simulink model "project"  (R2023b)
settings: Solver=VariableStepAuto  StartTime=0.0  StopTime=10.0  RelTol=1e-3
libraries: spsDCVoltageSourceLib x2, spsDCMachineLib x1, sps_lib x1
settings Model: Creator=yasha  LastModifiedBy=yasha

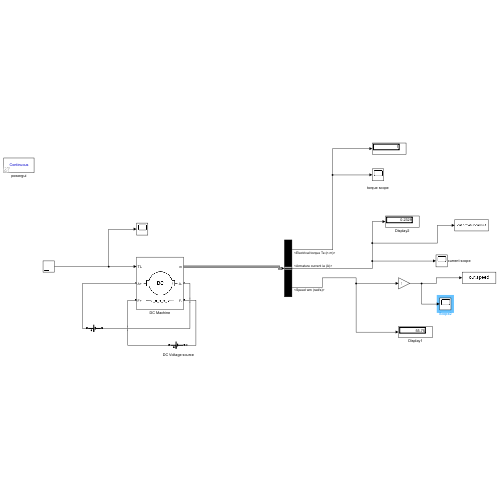
[thumbnail: Simulink's stored preview of the top-level diagram]
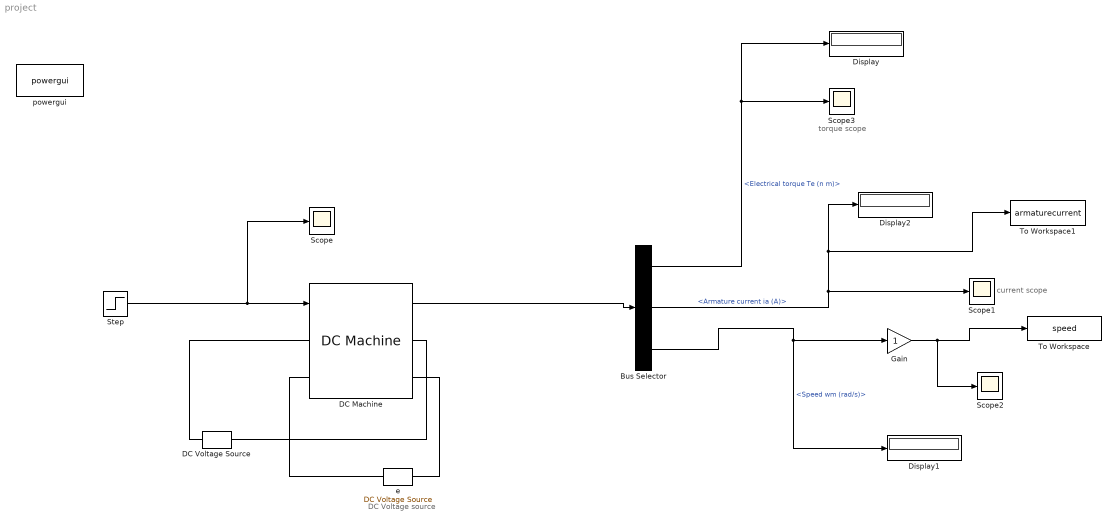
== system project ==
  note: DC Voltage source
  note: current scope
  note: torque scope
  Bus Selector : BusSelector  OutputSignals=Electrical torque Te (n m),Armature current ia (A),Speed wm (rad/s)
  DC Machine : spsDCMachineLib/DC Machine  PresetModel=No  MechanicalLoad=Torque TL  FieldType=Wound  ShowDetailedParameters=on  MeasurementBus=off  RLa=[2.581 0.028]  RLf="[ 53  156]"  Laf=0.9483  MachineConstant=Torque constant (N.m/A)  Ke=1.8  Kt=1.8  J=1  Bm=0  Tf=0  w0=1  Ifinit=4.52830188679245  TsPowergui=0  TsBlock=-1
  DC Voltage Source : spsDCVoltageSourceLib/DC Voltage Source  Amplitude=240  Measurements=None
  Display : Display
  Display1 : Display
  Display2 : Display
  Gain : Gain
  Scope{,1..3} (4 alike) : Scope
  Step : Step  SampleTime=0
  To Workspace : ToWorkspace  VariableName=speed  SaveFormat=Timeseries  SampleTime=-1
  To Workspace1 : ToWorkspace  VariableName=armaturecurrent  SaveFormat=Timeseries  SampleTime=-1
  e : spsDCVoltageSourceLib/DC Voltage Source  Amplitude=240  Measurements=Voltage
  powergui : sps_lib/powergui  Priority=1  SimulationMode=Continuous  SampleTime=50e-6  frequency=60  Iterations=50  frequencyindice=0  Pbase=100e6  ErrMax=1e-4  UnitsV=kV  UnitsW=MW  buscounter=0  FunctionMessages=off  echomessages=off  EnableUseOfTLC=off  CurrentSourceSwitches=off  DisableSnubberDevices=off  DisableRonSwitches=off  DisableVfSwitches=off  DisplayEquations=off  AutomaticDiscreteSolvers=off  SolverType=Tustin/Backward Euler (TBE)  Interpol=off  ExternalGateDelay=off  methode=off  Ts=100  x0status=blocks  SPID=on  SwTol=0  HookPort=off  NonlinearTolerance=1e-4  nMaxIteration=100  ContinueOnMaxIteration=off  RestoreLinks=warning  ResistiveCurrentMeasurement=off  Frange=[0:2:500]  Ylog=off  Xlog=on  ShowGrid=off  save=off  variable=ZData  structure=0  ZoomFFT=off  StartTime=0.0  cycles=1  DisplayStyle=1  fundamental=60  FreqAxis=off  MaxFrequency=1000  frequencyindicesteady=1  RmsSteady=1  display=off
  wires:
  Step/1 -> Scope/1, DC Machine/1
  DC Machine/1 -> Bus Selector/1
  Bus Selector/3 -> Gain/1, Display1/1  "<Speed wm (rad/s)>"
  Bus Selector/1 -> Display/1, Scope3/1  "<Electrical torque Te (n m)>"
  Bus Selector/2 -> To Workspace1/1, Display2/1, Scope1/1  "<Armature current ia (A)>"
  Gain/1 -> Scope2/1, To Workspace/1
  connections:
  DC Machine/LConn2 -- e/RConn1
  DC Machine/RConn2 -- e/LConn1
  DC Machine/LConn1 -- DC Voltage Source/RConn1
  DC Voltage Source/LConn1 -- DC Machine/RConn1
